simulink model "progetto3aSimulink"  (R2021a)
settings: Solver=VariableStepAuto  StartTime=0.0  StopTime=10  RelTol=1e-3
values from neighbouring files (symbols this model uses):
  A = [0 , 1; 0 , -(bb/(Mi*Ei*Ei+Ie))-(( (Ud*Mi*Ei*Ei)/(Mi*Ei*Ei+Ie) )*2*We) ]    [Progetto3a.m]    (also in Progetto4c.m = [0, 1; ((-gg*mm*ee)*cos(pi/2))/((mm*ee*ee+Ie)), -beta/(mm*ee; ProgettoGruppoAO.m; Progetto_Ada.m = [0, 1; ((-gg*mm*ee)*cos(pi/2))/((mm*ee*ee+Ie)), -beta/(mm*ee; Prova.m = [0, 1; 0, (bb/(Mi*Ei*Ei+Ie))-(( (Ud*Mi*Ei*Ei)/(Mi*Ei*Ei+Ie) )
  B = [0; 1/(Mi*Ei*Ei+Ie)]    [Progetto3a.m]    (also in Progetto4c.m = [0;1/(mm*ee*ee + Ie)]; ProgettoGruppoAO.m; Progetto_Ada.m = [0;1/(mm*ee*ee + Ie)]; Prova.m)
  C = [0 , 1]    [Progetto3a.m]    (also in Progetto4c.m = [0, 1]; ProgettoGruppoAO.m; Progetto_Ada.m = [0, 1]; Prova.m = [0, 1])
  den_r = d_r{1}    [Progetto3a.m]    (also in Progetto4c.m; ProgettoGruppoAO.m; Progetto_Ada.m; Prova.m)
  num_r = n_r{1}    [Progetto3a.m]    (also in Progetto4c.m; ProgettoGruppoAO.m; Progetto_Ada.m; Prova.m)
  omega_n = 100    [Progetto3a.m]    (also in Progetto4c.m = 120; ProgettoGruppoAO.m; Progetto_Ada.m = 120; Prova.m)
  u_e = 1110.7222    [Progetto3a.m]    (also in ProgettoGruppoAO.m)
  W = 5    [Progetto3a.m]    (also in Progetto4c.m = 4; ProgettoGruppoAO.m; Progetto_Ada.m = 4; Prova.m)
  x0 = [0,We]    [Progetto3a.m]    (also in Progetto4c.m = [0;0]; ProgettoGruppoAO.m = [teta_e,We]; Progetto_Ada.m = [0;0]; Prova.m = [teta_e,We])
  y_e = We    (= 1591.54943092)    [Progetto3a.m]    (also in ProgettoGruppoAO.m)
settings Model: Creator=Giacomo  LastModifiedBy=Giacomo

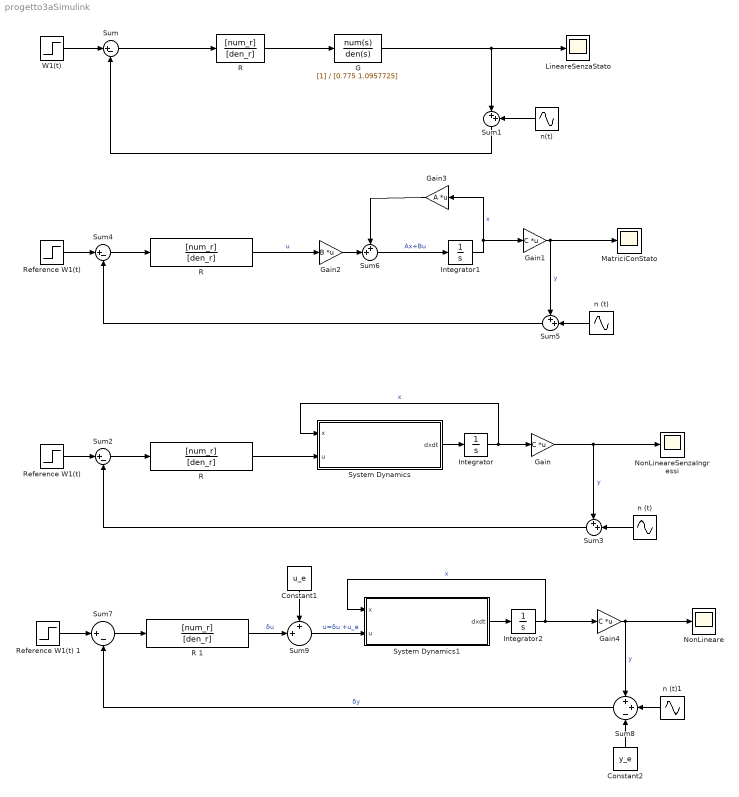
== system progetto3aSimulink ==
  Constant1 : Constant  Value=u_e
  Constant2 : Constant  Value=y_e
  G : TransferFcn  Denominator=[0.775 1.0957725]
  Gain : Gain  Gain=C  Multiplication=Matrix(K*u)
  Gain1 : Gain  Gain=C  Multiplication=Matrix(K*u)
  Gain2 : Gain  Gain=B  Multiplication=Matrix(K*u)
  Gain3 : Gain  Gain=A  Multiplication=Matrix(K*u)
  Gain4 : Gain  Gain=C  Multiplication=Matrix(K*u)
  Integrator : Integrator  InitialCondition=x0
  Integrator1 : Integrator  InitialCondition=[0, 0]
  Integrator2 : Integrator  InitialCondition=[0, 10000/(2*pi) + 800000]
  LineareSenzaStato : Scope
  MatriciConStato : Scope
  NonLineare : Scope
  NonLineareSenzaIngressi : Scope
  R : TransferFcn  Numerator=[num_r]  Denominator=[den_r]
  "R " : TransferFcn  Numerator=[num_r]  Denominator=[den_r]
  "R " : TransferFcn  Numerator=[num_r]  Denominator=[den_r]
  R 1 : TransferFcn  Numerator=[num_r]  Denominator=[den_r]
  "Reference W1(t) " : Step  After=W  SampleTime=0
  "Reference W1(t) " : Step  After=W  SampleTime=0
  Reference W1(t) 1 : Step  After=W  SampleTime=0
  Sum{,2,4,7} (4 alike) : Sum  Inputs=|+-
  Sum1 : Sum  Inputs=|++
  Sum{3,5..6,9} (4 alike) : Sum  Inputs=++|
  Sum8 : Sum  Inputs=++-
  System Dynamics : MATLAB Function  TreatAsAtomicUnit=on
  System Dynamics1 : MATLAB Function  TreatAsAtomicUnit=on
  W1(t) : Step  After=W  SampleTime=0
  n (t) : Sin  Amplitude=0.02  Frequency=omega_n  SampleTime=0
  "n (t) " : Sin  Amplitude=0.02  Frequency=omega_n  SampleTime=0
  n (t)1 : Sin  Amplitude=0.02  Frequency=omega_n  SampleTime=0
  n(t) : Sin  Amplitude=0.02  Frequency=omega_n  SampleTime=0  VectorParams1D=off
  wires:
  Sum1/1 -> Sum/2
  W1(t)/1 -> Sum/1
  G/1 -> LineareSenzaStato/1, Sum1/1
  R/1 -> G/1
  n(t)/1 -> Sum1/2
  Sum/1 -> R/1
  Sum6/1 -> Integrator1/1  "Ax+Bu"
  Gain3/1 -> Sum6/1
  "Reference W1(t) "/1 -> Sum4/1
  Gain2/1 -> Sum6/2
  "n (t) "/1 -> Sum5/2
  Sum4/1 -> "R "/1
  Gain1/1 -> Sum5/1, MatriciConStato/1  "y"
  Integrator1/1 -> Gain1/1, Gain3/1  "x"
  "R "/1 -> Gain2/1  "u"
  Sum5/1 -> Sum4/2
  n (t)/1 -> Sum3/2
  "Reference W1(t) "/1 -> Sum2/1
  Sum3/1 -> Sum2/2
  System Dynamics/1(dxdt) -> Integrator/1
  Gain/1 -> NonLineareSenzaIngressi/1, Sum3/1  "y"
  Integrator/1 -> System Dynamics/1(x), Gain/1  "x"
  Sum2/1 -> "R "/1
  "R "/1 -> System Dynamics/2(u)
  R 1/1 -> Sum9/2  "δu"
  Gain4/1 -> NonLineare/1, Sum8/1  "y"
  Sum7/1 -> R 1/1
  Reference W1(t) 1/1 -> Sum7/1
  System Dynamics1/1(dxdt) -> Integrator2/1
  Sum8/1 -> Sum7/2  "δy"
  n (t)1/1 -> Sum8/2
  Integrator2/1 -> System Dynamics1/1(x), Gain4/1  "x"
  Constant1/1 -> Sum9/1
  Constant2/1 -> Sum8/3
  Sum9/1 -> System Dynamics1/2(u)  "u=δu +u_e"

== matlab function progetto3aSimulink/System Dynamics ==
  data: x input; u input; dxdt output
function dxdt = systemDynamics(x,u)
bb=0.3;
Ud=0.01;
Mi=0.1;
Ei=0.5;
Ie=0.75;

dx1dt = x(2);
dx2dt =( -bb*x(2)- (Ud*Mi*(Ei^2)*(x(2)^2) ) + u ) / (Mi*Ei*Ei+Ie);
%dxdt = [dx1dt; dx2dt; dx3dt;...;dxndt];
dxdt = [dx1dt; dx2dt];

== matlab function progetto3aSimulink/System Dynamics1 ==
  data: x input; u input; dxdt output
function dxdt = systemDynamics(x,u)
bb=0.3;
Ud=0.01;
Mi=0.1;
Ei=0.5;
Ie=0.75;
%Ue=-477.06;

dx1dt = x(2);
dx2dt =( -bb*x(2)- (Ud*Mi*Ei*Ei*x(2)*x(2) ) + u ) / (Mi*Ei*Ei+Ie);
%dxdt = [dx1dt; dx2dt; dx3dt;...;dxndt];
dxdt = [dx1dt; dx2dt];
